simulink library "inverter_leg"  (R2018a)
settings: Solver=VariableStepAuto  StartTime=0.0  StopTime=10.0  RelTol=1e-3
libraries: powerlib x8
settings Model: Creator=AL-MOSTAFA  LastModifiedBy=AL-MOSTAFA

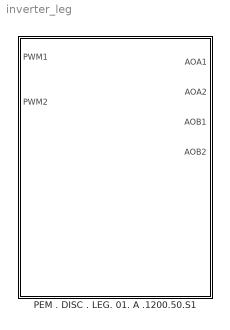
== system inverter_leg ==
  PEM . DISC . LEG. 01. A .1200.50.S1 : Subsystem

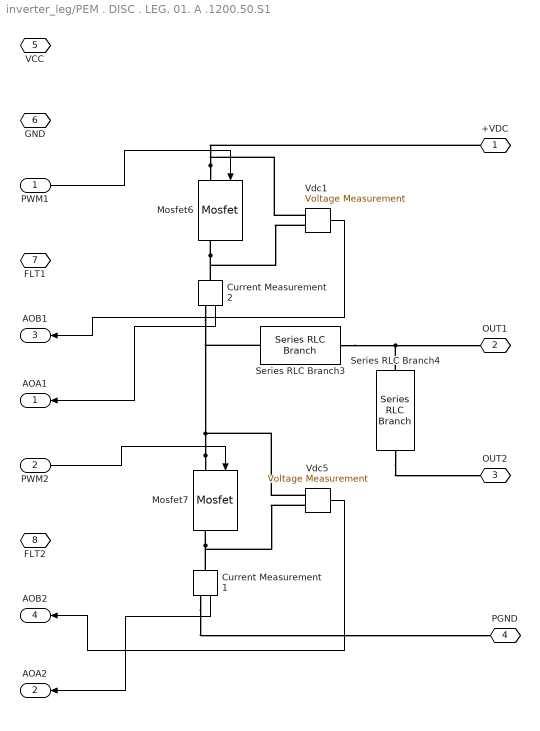
== system inverter_leg/PEM . DISC . LEG. 01. A .1200.50.S1 ==
  PWM1 : Inport
  PWM2 : Inport  Port=2
  Current Measurement1 : powerlib/Measurements/Current Measurement  PhasorSimulation=off  OutputType=Complex  PSBequivalent=0
  Current Measurement2 : powerlib/Measurements/Current Measurement  PhasorSimulation=off  OutputType=Complex  PSBequivalent=0
  Mosfet6 : powerlib/Power Electronics/Mosfet  Ron=0.1  Lon=0  Rd=0.01  Vfd=0  IC=0  Rs=1e5  Cs=inf  Measurements=on
  Mosfet7 : powerlib/Power Electronics/Mosfet  Ron=0.1  Lon=0  Rd=0.01  Vfd=0  IC=0  Rs=1e5  Cs=inf  Measurements=on
  Series RLC Branch3 : powerlib/Elements/Series RLC Branch  LConnTagsString=__new0  RConnTagsString=__new0  BranchType=L  Resistance=10  Inductance=1e-2  SetiL0=off  InitialCurrent=0  Capacitance=10^-3  Setx0=off  InitialVoltage=0  Measurements=None
  Series RLC Branch4 : powerlib/Elements/Series RLC Branch  LConnTagsString=__new0  RConnTagsString=__new0  BranchType=C  Resistance=10  Inductance=1e-2  SetiL0=off  InitialCurrent=0  Capacitance=10^-3  Setx0=off  InitialVoltage=0  Measurements=None
  Vdc1 : powerlib/Measurements/Voltage Measurement  PhasorSimulation=off  OutputType=Complex  PSBequivalent=0
  Vdc5 : powerlib/Measurements/Voltage Measurement  PhasorSimulation=off  OutputType=Complex  PSBequivalent=0
  +VDC : PMIOPort  Side=Right
  OUT1 : PMIOPort  Port=2  Side=Right
  OUT2 : PMIOPort  Port=3  Side=Right
  PGND : PMIOPort  Port=4  Side=Right
  VCC : PMIOPort  Port=5  Side=Left
  GND : PMIOPort  Port=6  Side=Left
  FLT1 : PMIOPort  Port=7  Side=Left
  FLT2 : PMIOPort  Port=8  Side=Left
  AOA1 : Outport
  AOA2 : Outport  Port=2
  AOB1 : Outport  Port=3
  AOB2 : Outport  Port=4
  wires:
  PWM1/1 -> Mosfet6/1
  PWM2/1 -> Mosfet7/1
  Current Measurement2/1 -> AOA1/1
  Current Measurement1/1 -> AOA2/1
  Vdc1/1 -> AOB1/1
  Vdc5/1 -> AOB2/1
  connections:
  Mosfet6/LConn1 -- +VDC/RConn1 -- Vdc1/LConn1
  Series RLC Branch4/RConn1 -- OUT2/RConn1
  Series RLC Branch4/LConn1 -- Series RLC Branch3/RConn1 -- OUT1/RConn1
  Mosfet6/RConn1 -- Current Measurement2/LConn1 -- Vdc1/LConn2
  Mosfet7/LConn1 -- Series RLC Branch3/LConn1 -- Current Measurement2/RConn1 -- Vdc5/LConn1
  Mosfet7/RConn1 -- Current Measurement1/LConn1 -- Vdc5/LConn2
  Current Measurement1/RConn1 -- PGND/RConn1
